simulink model "GIT_AUTO_Model_Example"  (R2019b)
settings: Solver=FixedStepDiscrete  StartTime=0.0  StopTime=10  FixedStep=0.01  RelTol=1e-3  EnableMultiTasking=on
InitFcn:
  | clear mex;
undefined symbols (not defined in the file): asbcbaseini_C, ibatini_C, k_icalpl_C, scsocini_C, stopengstmode_C, t_bmaxini_C, t_bminini_C, t_vminddstr_C, TSB_Coulomb_float, TSB_Dc_float, TSB_Pwr_float, TSB_R_float, TSB_Soc, TSB_Tbatt, TSB_Tbatt_float, TSB_value_float, TSB_Volt_float, v_bcini_C, v_bcmaxini_C
libraries: Utility_Block_Library x22, AMO_Block_Library x2
(part 3 of 5)

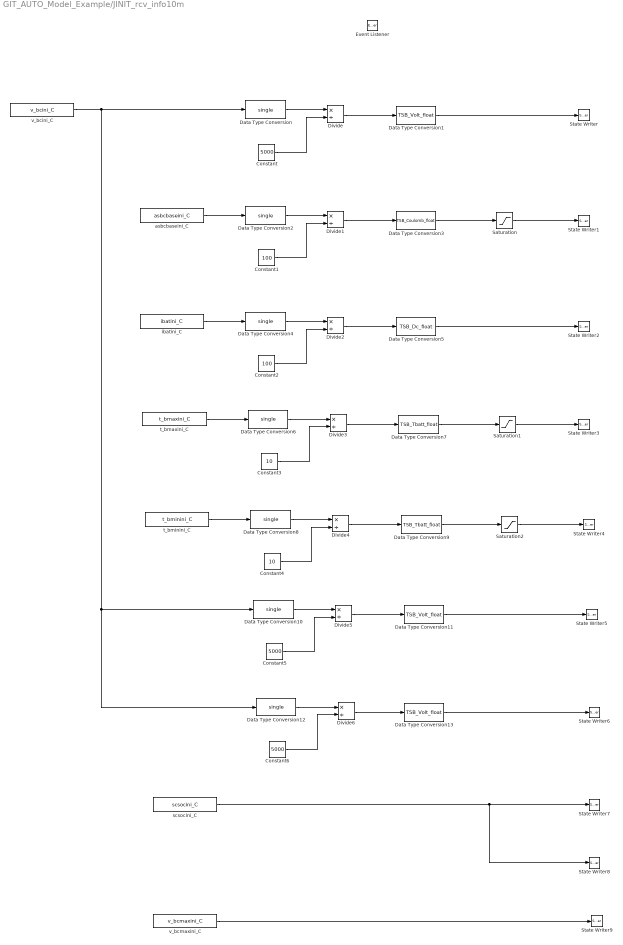
== system GIT_AUTO_Model_Example/JINIT_rcv_info10m ==
  Constant : Constant  Tag=#AMO_Lib  Value=5000  OutDataTypeStr=single
      settings: AttributesFormatString=%<Tag>\nOutDataType = %<OutDataTypeStr>
  Constant1 : Constant  Tag=#AMO_Lib  Value=100  OutDataTypeStr=single
      settings: AttributesFormatString=%<Tag>\nOutDataType = %<OutDataTypeStr>
  Constant2 : Constant  Tag=#AMO_Lib  Value=100  OutDataTypeStr=single
      settings: AttributesFormatString=%<Tag>\nOutDataType = %<OutDataTypeStr>
  Constant3 : Constant  Tag=#AMO_Lib  Value=10  OutDataTypeStr=single
      settings: AttributesFormatString=%<Tag>\nOutDataType = %<OutDataTypeStr>
  Constant4 : Constant  Tag=#AMO_Lib  Value=10  OutDataTypeStr=single
      settings: AttributesFormatString=%<Tag>\nOutDataType = %<OutDataTypeStr>
  Constant5 : Constant  Tag=#AMO_Lib  Value=5000  OutDataTypeStr=single
      settings: AttributesFormatString=%<Tag>\nOutDataType = %<OutDataTypeStr>
  Constant6 : Constant  Tag=#AMO_Lib  Value=5000  OutDataTypeStr=single
      settings: AttributesFormatString=%<Tag>\nOutDataType = %<OutDataTypeStr>
  Data Type Conversion : DataTypeConversion  Tag=#AMO_Lib  OutMin=OutMin  OutMax=OutMax  OutDataTypeStr=single  ConvertRealWorld=Stored Integer (SI)  SampleTime=SampleTime  SaturateOnIntegerOverflow=on  RndMeth=Zero  mask{OutMin=[], OutMax=[], OutDataTypeStr=single, LockScale=off, ConvertRealWorld=Stored Integer (SI), RndMeth=Zero, SaturateOnIntegerOverflow=on, SampleTime=-1}
      mask prompts: OutMin "Simulink:blkprm_prompts:OutputDesignMin"; OutMax "Simulink:blkprm_prompts:OutputDesignMax"; OutDataTypeStr "Simulink:blkprm_prompts:OUTPUT_UNIFIEDDATATYPE"; LockScale "Simulink:blkprm_prompts:LockScale"; ConvertRealWorld "Simulink:blkprm_prompts:DtypeCnvInputOutputValue"; RndMeth "Simulink:blkprm_prompts:SPP_RndMeth_ID"; SaturateOnIntegerOverflow "Simulink:blkprm_prompts:AllBlksSaturate"; SampleTime "Simulink:blkprm_prompts:AllBlksSampleTime"
      mask help:
      | 入力を出力のデータ型とスケーリングに変換します。
      |
      | この変換には 2 つの目的があります。1 つは入力と出力の実際値を等しくすることです。もう 1 つは入力と出力の整数格納値を等しくすることです。オーバーフローと量子化誤差があると、この目的を完全に達成することができません。
      settings: AttributesFormatString=%<Tag>\nOutDataType = %<OutDataTypeStr>
      mask TypeOptions OutMin: OutMin
      mask TypeOptions OutMax: OutMax
      mask TypeOptions OutDataTypeStr: OutDataTypeStr
      mask TypeOptions LockScale: LockScale
      mask TypeOptions ConvertRealWorld: ConvertRealWorld
      mask TypeOptions RndMeth: RndMeth
      mask TypeOptions SaturateOnIntegerOverflow: SaturateOnIntegerOverflow
      mask TypeOptions SampleTime: SampleTime
      mask DialogControl OutMin Prompt: 出力の最小値:
      mask DialogControl OutMax Prompt: 出力の最大値:
      mask DialogControl OutDataTypeStr Prompt: 出力データ型:
      mask DialogControl LockScale Prompt: 固定小数点ツールによる変更に対して出力データ型の設定をロックする
      mask DialogControl ConvertRealWorld Prompt: 等価な値をもつ入力と出力:
      mask DialogControl RndMeth Prompt: 整数丸めモード:
      mask DialogControl SaturateOnIntegerOverflow Prompt: 整数オーバーフローで飽和
      mask DialogControl SampleTime Prompt: サンプル時間 (継承は -1):
  Data Type Conversion1 : DataTypeConversion  Tag=#AMO_Lib  OutMin=OutMin  OutMax=OutMax  OutDataTypeStr=TSB_Volt_float  SampleTime=SampleTime  SaturateOnIntegerOverflow=on  RndMeth=Zero  mask{OutMin=[], OutMax=[], OutDataTypeStr=TSB_Volt_float, LockScale=off, ConvertRealWorld=Real World Value (RWV), RndMeth=Zero, SaturateOnIntegerOverflow=on, SampleTime=-1}
      mask prompts: OutMin "Simulink:blkprm_prompts:OutputDesignMin"; OutMax "Simulink:blkprm_prompts:OutputDesignMax"; OutDataTypeStr "Simulink:blkprm_prompts:OUTPUT_UNIFIEDDATATYPE"; LockScale "Simulink:blkprm_prompts:LockScale"; ConvertRealWorld "Simulink:blkprm_prompts:DtypeCnvInputOutputValue"; RndMeth "Simulink:blkprm_prompts:SPP_RndMeth_ID"; SaturateOnIntegerOverflow "Simulink:blkprm_prompts:AllBlksSaturate"; SampleTime "Simulink:blkprm_prompts:AllBlksSampleTime"
      mask help:
      | 入力を出力のデータ型とスケーリングに変換します。
      |
      | この変換には 2 つの目的があります。1 つは入力と出力の実際値を等しくすることです。もう 1 つは入力と出力の整数格納値を等しくすることです。オーバーフローと量子化誤差があると、この目的を完全に達成することができません。
      settings: AttributesFormatString=%<Tag>\nOutDataType = %<OutDataTypeStr>
      mask TypeOptions OutMin: OutMin
      mask TypeOptions OutMax: OutMax
      mask TypeOptions OutDataTypeStr: OutDataTypeStr
      mask TypeOptions LockScale: LockScale
      mask TypeOptions ConvertRealWorld: ConvertRealWorld
      mask TypeOptions RndMeth: RndMeth
      mask TypeOptions SaturateOnIntegerOverflow: SaturateOnIntegerOverflow
      mask TypeOptions SampleTime: SampleTime
      mask DialogControl OutMin Prompt: 出力の最小値:
      mask DialogControl OutMax Prompt: 出力の最大値:
      mask DialogControl OutDataTypeStr Prompt: 出力データ型:
      mask DialogControl LockScale Prompt: 固定小数点ツールによる変更に対して出力データ型の設定をロックする
      mask DialogControl ConvertRealWorld Prompt: 等価な値をもつ入力と出力:
      mask DialogControl RndMeth Prompt: 整数丸めモード:
      mask DialogControl SaturateOnIntegerOverflow Prompt: 整数オーバーフローで飽和
      mask DialogControl SampleTime Prompt: サンプル時間 (継承は -1):
  Data Type Conversion10 : DataTypeConversion  Tag=#AMO_Lib  OutMin=OutMin  OutMax=OutMax  OutDataTypeStr=single  ConvertRealWorld=Stored Integer (SI)  SampleTime=SampleTime  SaturateOnIntegerOverflow=on  RndMeth=Zero  mask{OutMin=[], OutMax=[], OutDataTypeStr=single, LockScale=off, ConvertRealWorld=Stored Integer (SI), RndMeth=Zero, SaturateOnIntegerOverflow=on, SampleTime=-1}
      mask prompts: OutMin "Simulink:blkprm_prompts:OutputDesignMin"; OutMax "Simulink:blkprm_prompts:OutputDesignMax"; OutDataTypeStr "Simulink:blkprm_prompts:OUTPUT_UNIFIEDDATATYPE"; LockScale "Simulink:blkprm_prompts:LockScale"; ConvertRealWorld "Simulink:blkprm_prompts:DtypeCnvInputOutputValue"; RndMeth "Simulink:blkprm_prompts:SPP_RndMeth_ID"; SaturateOnIntegerOverflow "Simulink:blkprm_prompts:AllBlksSaturate"; SampleTime "Simulink:blkprm_prompts:AllBlksSampleTime"
      mask help:
      | 入力を出力のデータ型とスケーリングに変換します。
      |
      | この変換には 2 つの目的があります。1 つは入力と出力の実際値を等しくすることです。もう 1 つは入力と出力の整数格納値を等しくすることです。オーバーフローと量子化誤差があると、この目的を完全に達成することができません。
      settings: AttributesFormatString=%<Tag>\nOutDataType = %<OutDataTypeStr>
      mask TypeOptions OutMin: OutMin
      mask TypeOptions OutMax: OutMax
      mask TypeOptions OutDataTypeStr: OutDataTypeStr
      mask TypeOptions LockScale: LockScale
      mask TypeOptions ConvertRealWorld: ConvertRealWorld
      mask TypeOptions RndMeth: RndMeth
      mask TypeOptions SaturateOnIntegerOverflow: SaturateOnIntegerOverflow
      mask TypeOptions SampleTime: SampleTime
      mask DialogControl OutMin Prompt: 出力の最小値:
      mask DialogControl OutMax Prompt: 出力の最大値:
      mask DialogControl OutDataTypeStr Prompt: 出力データ型:
      mask DialogControl LockScale Prompt: 固定小数点ツールによる変更に対して出力データ型の設定をロックする
      mask DialogControl ConvertRealWorld Prompt: 等価な値をもつ入力と出力:
      mask DialogControl RndMeth Prompt: 整数丸めモード:
      mask DialogControl SaturateOnIntegerOverflow Prompt: 整数オーバーフローで飽和
      mask DialogControl SampleTime Prompt: サンプル時間 (継承は -1):
  Data Type Conversion11 : DataTypeConversion  Tag=#AMO_Lib  OutMin=OutMin  OutMax=OutMax  OutDataTypeStr=TSB_Volt_float  SampleTime=SampleTime  SaturateOnIntegerOverflow=on  RndMeth=Zero  mask{OutMin=[], OutMax=[], OutDataTypeStr=TSB_Volt_float, LockScale=off, ConvertRealWorld=Real World Value (RWV), RndMeth=Zero, SaturateOnIntegerOverflow=on, SampleTime=-1}
      mask prompts: OutMin "Simulink:blkprm_prompts:OutputDesignMin"; OutMax "Simulink:blkprm_prompts:OutputDesignMax"; OutDataTypeStr "Simulink:blkprm_prompts:OUTPUT_UNIFIEDDATATYPE"; LockScale "Simulink:blkprm_prompts:LockScale"; ConvertRealWorld "Simulink:blkprm_prompts:DtypeCnvInputOutputValue"; RndMeth "Simulink:blkprm_prompts:SPP_RndMeth_ID"; SaturateOnIntegerOverflow "Simulink:blkprm_prompts:AllBlksSaturate"; SampleTime "Simulink:blkprm_prompts:AllBlksSampleTime"
      mask help:
      | 入力を出力のデータ型とスケーリングに変換します。
      |
      | この変換には 2 つの目的があります。1 つは入力と出力の実際値を等しくすることです。もう 1 つは入力と出力の整数格納値を等しくすることです。オーバーフローと量子化誤差があると、この目的を完全に達成することができません。
      settings: AttributesFormatString=%<Tag>\nOutDataType = %<OutDataTypeStr>
      mask TypeOptions OutMin: OutMin
      mask TypeOptions OutMax: OutMax
      mask TypeOptions OutDataTypeStr: OutDataTypeStr
      mask TypeOptions LockScale: LockScale
      mask TypeOptions ConvertRealWorld: ConvertRealWorld
      mask TypeOptions RndMeth: RndMeth
      mask TypeOptions SaturateOnIntegerOverflow: SaturateOnIntegerOverflow
      mask TypeOptions SampleTime: SampleTime
      mask DialogControl OutMin Prompt: 出力の最小値:
      mask DialogControl OutMax Prompt: 出力の最大値:
      mask DialogControl OutDataTypeStr Prompt: 出力データ型:
      mask DialogControl LockScale Prompt: 固定小数点ツールによる変更に対して出力データ型の設定をロックする
      mask DialogControl ConvertRealWorld Prompt: 等価な値をもつ入力と出力:
      mask DialogControl RndMeth Prompt: 整数丸めモード:
      mask DialogControl SaturateOnIntegerOverflow Prompt: 整数オーバーフローで飽和
      mask DialogControl SampleTime Prompt: サンプル時間 (継承は -1):
  Data Type Conversion12 : DataTypeConversion  Tag=#AMO_Lib  OutMin=OutMin  OutMax=OutMax  OutDataTypeStr=single  ConvertRealWorld=Stored Integer (SI)  SampleTime=SampleTime  SaturateOnIntegerOverflow=on  RndMeth=Zero  mask{OutMin=[], OutMax=[], OutDataTypeStr=single, LockScale=off, ConvertRealWorld=Stored Integer (SI), RndMeth=Zero, SaturateOnIntegerOverflow=on, SampleTime=-1}
      mask prompts: OutMin "Simulink:blkprm_prompts:OutputDesignMin"; OutMax "Simulink:blkprm_prompts:OutputDesignMax"; OutDataTypeStr "Simulink:blkprm_prompts:OUTPUT_UNIFIEDDATATYPE"; LockScale "Simulink:blkprm_prompts:LockScale"; ConvertRealWorld "Simulink:blkprm_prompts:DtypeCnvInputOutputValue"; RndMeth "Simulink:blkprm_prompts:SPP_RndMeth_ID"; SaturateOnIntegerOverflow "Simulink:blkprm_prompts:AllBlksSaturate"; SampleTime "Simulink:blkprm_prompts:AllBlksSampleTime"
      mask help:
      | 入力を出力のデータ型とスケーリングに変換します。
      |
      | この変換には 2 つの目的があります。1 つは入力と出力の実際値を等しくすることです。もう 1 つは入力と出力の整数格納値を等しくすることです。オーバーフローと量子化誤差があると、この目的を完全に達成することができません。
      settings: AttributesFormatString=%<Tag>\nOutDataType = %<OutDataTypeStr>
      mask TypeOptions OutMin: OutMin
      mask TypeOptions OutMax: OutMax
      mask TypeOptions OutDataTypeStr: OutDataTypeStr
      mask TypeOptions LockScale: LockScale
      mask TypeOptions ConvertRealWorld: ConvertRealWorld
      mask TypeOptions RndMeth: RndMeth
      mask TypeOptions SaturateOnIntegerOverflow: SaturateOnIntegerOverflow
      mask TypeOptions SampleTime: SampleTime
      mask DialogControl OutMin Prompt: 出力の最小値:
      mask DialogControl OutMax Prompt: 出力の最大値:
      mask DialogControl OutDataTypeStr Prompt: 出力データ型:
      mask DialogControl LockScale Prompt: 固定小数点ツールによる変更に対して出力データ型の設定をロックする
      mask DialogControl ConvertRealWorld Prompt: 等価な値をもつ入力と出力:
      mask DialogControl RndMeth Prompt: 整数丸めモード:
      mask DialogControl SaturateOnIntegerOverflow Prompt: 整数オーバーフローで飽和
      mask DialogControl SampleTime Prompt: サンプル時間 (継承は -1):
  Data Type Conversion13 : DataTypeConversion  Tag=#AMO_Lib  OutMin=OutMin  OutMax=OutMax  OutDataTypeStr=TSB_Volt_float  SampleTime=SampleTime  SaturateOnIntegerOverflow=on  RndMeth=Zero  mask{OutMin=[], OutMax=[], OutDataTypeStr=TSB_Volt_float, LockScale=off, ConvertRealWorld=Real World Value (RWV), RndMeth=Zero, SaturateOnIntegerOverflow=on, SampleTime=-1}
      mask prompts: OutMin "Simulink:blkprm_prompts:OutputDesignMin"; OutMax "Simulink:blkprm_prompts:OutputDesignMax"; OutDataTypeStr "Simulink:blkprm_prompts:OUTPUT_UNIFIEDDATATYPE"; LockScale "Simulink:blkprm_prompts:LockScale"; ConvertRealWorld "Simulink:blkprm_prompts:DtypeCnvInputOutputValue"; RndMeth "Simulink:blkprm_prompts:SPP_RndMeth_ID"; SaturateOnIntegerOverflow "Simulink:blkprm_prompts:AllBlksSaturate"; SampleTime "Simulink:blkprm_prompts:AllBlksSampleTime"
      mask help:
      | 入力を出力のデータ型とスケーリングに変換します。
      |
      | この変換には 2 つの目的があります。1 つは入力と出力の実際値を等しくすることです。もう 1 つは入力と出力の整数格納値を等しくすることです。オーバーフローと量子化誤差があると、この目的を完全に達成することができません。
      settings: AttributesFormatString=%<Tag>\nOutDataType = %<OutDataTypeStr>
      mask TypeOptions OutMin: OutMin
      mask TypeOptions OutMax: OutMax
      mask TypeOptions OutDataTypeStr: OutDataTypeStr
      mask TypeOptions LockScale: LockScale
      mask TypeOptions ConvertRealWorld: ConvertRealWorld
      mask TypeOptions RndMeth: RndMeth
      mask TypeOptions SaturateOnIntegerOverflow: SaturateOnIntegerOverflow
      mask TypeOptions SampleTime: SampleTime
      mask DialogControl OutMin Prompt: 出力の最小値:
      mask DialogControl OutMax Prompt: 出力の最大値:
      mask DialogControl OutDataTypeStr Prompt: 出力データ型:
      mask DialogControl LockScale Prompt: 固定小数点ツールによる変更に対して出力データ型の設定をロックする
      mask DialogControl ConvertRealWorld Prompt: 等価な値をもつ入力と出力:
      mask DialogControl RndMeth Prompt: 整数丸めモード:
      mask DialogControl SaturateOnIntegerOverflow Prompt: 整数オーバーフローで飽和
      mask DialogControl SampleTime Prompt: サンプル時間 (継承は -1):
  Data Type Conversion2 : DataTypeConversion  Tag=#AMO_Lib  OutMin=OutMin  OutMax=OutMax  OutDataTypeStr=single  ConvertRealWorld=Stored Integer (SI)  SampleTime=SampleTime  SaturateOnIntegerOverflow=on  RndMeth=Zero  mask{OutMin=[], OutMax=[], OutDataTypeStr=single, LockScale=off, ConvertRealWorld=Stored Integer (SI), RndMeth=Zero, SaturateOnIntegerOverflow=on, SampleTime=-1}
      mask prompts: OutMin "Simulink:blkprm_prompts:OutputDesignMin"; OutMax "Simulink:blkprm_prompts:OutputDesignMax"; OutDataTypeStr "Simulink:blkprm_prompts:OUTPUT_UNIFIEDDATATYPE"; LockScale "Simulink:blkprm_prompts:LockScale"; ConvertRealWorld "Simulink:blkprm_prompts:DtypeCnvInputOutputValue"; RndMeth "Simulink:blkprm_prompts:SPP_RndMeth_ID"; SaturateOnIntegerOverflow "Simulink:blkprm_prompts:AllBlksSaturate"; SampleTime "Simulink:blkprm_prompts:AllBlksSampleTime"
      mask help:
      | 入力を出力のデータ型とスケーリングに変換します。
      |
      | この変換には 2 つの目的があります。1 つは入力と出力の実際値を等しくすることです。もう 1 つは入力と出力の整数格納値を等しくすることです。オーバーフローと量子化誤差があると、この目的を完全に達成することができません。
      settings: AttributesFormatString=%<Tag>\nOutDataType = %<OutDataTypeStr>
      mask TypeOptions OutMin: OutMin
      mask TypeOptions OutMax: OutMax
      mask TypeOptions OutDataTypeStr: OutDataTypeStr
      mask TypeOptions LockScale: LockScale
      mask TypeOptions ConvertRealWorld: ConvertRealWorld
      mask TypeOptions RndMeth: RndMeth
      mask TypeOptions SaturateOnIntegerOverflow: SaturateOnIntegerOverflow
      mask TypeOptions SampleTime: SampleTime
      mask DialogControl OutMin Prompt: 出力の最小値:
      mask DialogControl OutMax Prompt: 出力の最大値:
      mask DialogControl OutDataTypeStr Prompt: 出力データ型:
      mask DialogControl LockScale Prompt: 固定小数点ツールによる変更に対して出力データ型の設定をロックする
      mask DialogControl ConvertRealWorld Prompt: 等価な値をもつ入力と出力:
      mask DialogControl RndMeth Prompt: 整数丸めモード:
      mask DialogControl SaturateOnIntegerOverflow Prompt: 整数オーバーフローで飽和
      mask DialogControl SampleTime Prompt: サンプル時間 (継承は -1):
  Data Type Conversion3 : DataTypeConversion  Tag=#AMO_Lib  OutMin=OutMin  OutMax=OutMax  OutDataTypeStr=TSB_Coulomb_float  SampleTime=SampleTime  SaturateOnIntegerOverflow=on  RndMeth=Zero  mask{OutMin=[], OutMax=[], OutDataTypeStr=TSB_Coulomb_float, LockScale=off, ConvertRealWorld=Real World Value (RWV), RndMeth=Zero, SaturateOnIntegerOverflow=on, SampleTime=-1}
      mask prompts: OutMin "Simulink:blkprm_prompts:OutputDesignMin"; OutMax "Simulink:blkprm_prompts:OutputDesignMax"; OutDataTypeStr "Simulink:blkprm_prompts:OUTPUT_UNIFIEDDATATYPE"; LockScale "Simulink:blkprm_prompts:LockScale"; ConvertRealWorld "Simulink:blkprm_prompts:DtypeCnvInputOutputValue"; RndMeth "Simulink:blkprm_prompts:SPP_RndMeth_ID"; SaturateOnIntegerOverflow "Simulink:blkprm_prompts:AllBlksSaturate"; SampleTime "Simulink:blkprm_prompts:AllBlksSampleTime"
      mask help:
      | 入力を出力のデータ型とスケーリングに変換します。
      |
      | この変換には 2 つの目的があります。1 つは入力と出力の実際値を等しくすることです。もう 1 つは入力と出力の整数格納値を等しくすることです。オーバーフローと量子化誤差があると、この目的を完全に達成することができません。
      settings: AttributesFormatString=%<Tag>\nOutDataType = %<OutDataTypeStr>
      mask TypeOptions OutMin: OutMin
      mask TypeOptions OutMax: OutMax
      mask TypeOptions OutDataTypeStr: OutDataTypeStr
      mask TypeOptions LockScale: LockScale
      mask TypeOptions ConvertRealWorld: ConvertRealWorld
      mask TypeOptions RndMeth: RndMeth
      mask TypeOptions SaturateOnIntegerOverflow: SaturateOnIntegerOverflow
      mask TypeOptions SampleTime: SampleTime
      mask DialogControl OutMin Prompt: 出力の最小値:
      mask DialogControl OutMax Prompt: 出力の最大値:
      mask DialogControl OutDataTypeStr Prompt: 出力データ型:
      mask DialogControl LockScale Prompt: 固定小数点ツールによる変更に対して出力データ型の設定をロックする
      mask DialogControl ConvertRealWorld Prompt: 等価な値をもつ入力と出力:
      mask DialogControl RndMeth Prompt: 整数丸めモード:
      mask DialogControl SaturateOnIntegerOverflow Prompt: 整数オーバーフローで飽和
      mask DialogControl SampleTime Prompt: サンプル時間 (継承は -1):
  Data Type Conversion4 : DataTypeConversion  Tag=#AMO_Lib  OutMin=OutMin  OutMax=OutMax  OutDataTypeStr=single  ConvertRealWorld=Stored Integer (SI)  SampleTime=SampleTime  SaturateOnIntegerOverflow=on  RndMeth=Zero  mask{OutMin=[], OutMax=[], OutDataTypeStr=single, LockScale=off, ConvertRealWorld=Stored Integer (SI), RndMeth=Zero, SaturateOnIntegerOverflow=on, SampleTime=-1}
      mask prompts: OutMin "Simulink:blkprm_prompts:OutputDesignMin"; OutMax "Simulink:blkprm_prompts:OutputDesignMax"; OutDataTypeStr "Simulink:blkprm_prompts:OUTPUT_UNIFIEDDATATYPE"; LockScale "Simulink:blkprm_prompts:LockScale"; ConvertRealWorld "Simulink:blkprm_prompts:DtypeCnvInputOutputValue"; RndMeth "Simulink:blkprm_prompts:SPP_RndMeth_ID"; SaturateOnIntegerOverflow "Simulink:blkprm_prompts:AllBlksSaturate"; SampleTime "Simulink:blkprm_prompts:AllBlksSampleTime"
      mask help:
      | 入力を出力のデータ型とスケーリングに変換します。
      |
      | この変換には 2 つの目的があります。1 つは入力と出力の実際値を等しくすることです。もう 1 つは入力と出力の整数格納値を等しくすることです。オーバーフローと量子化誤差があると、この目的を完全に達成することができません。
      settings: AttributesFormatString=%<Tag>\nOutDataType = %<OutDataTypeStr>
      mask TypeOptions OutMin: OutMin
      mask TypeOptions OutMax: OutMax
      mask TypeOptions OutDataTypeStr: OutDataTypeStr
      mask TypeOptions LockScale: LockScale
      mask TypeOptions ConvertRealWorld: ConvertRealWorld
      mask TypeOptions RndMeth: RndMeth
      mask TypeOptions SaturateOnIntegerOverflow: SaturateOnIntegerOverflow
      mask TypeOptions SampleTime: SampleTime
      mask DialogControl OutMin Prompt: 出力の最小値:
      mask DialogControl OutMax Prompt: 出力の最大値:
      mask DialogControl OutDataTypeStr Prompt: 出力データ型:
      mask DialogControl LockScale Prompt: 固定小数点ツールによる変更に対して出力データ型の設定をロックする
      mask DialogControl ConvertRealWorld Prompt: 等価な値をもつ入力と出力:
      mask DialogControl RndMeth Prompt: 整数丸めモード:
      mask DialogControl SaturateOnIntegerOverflow Prompt: 整数オーバーフローで飽和
      mask DialogControl SampleTime Prompt: サンプル時間 (継承は -1):
  Data Type Conversion5 : DataTypeConversion  Tag=#AMO_Lib  OutMin=OutMin  OutMax=OutMax  OutDataTypeStr=TSB_Dc_float  SampleTime=SampleTime  SaturateOnIntegerOverflow=on  RndMeth=Zero  mask{OutMin=[], OutMax=[], OutDataTypeStr=TSB_Dc_float, LockScale=off, ConvertRealWorld=Real World Value (RWV), RndMeth=Zero, SaturateOnIntegerOverflow=on, SampleTime=-1}
      mask prompts: OutMin "Simulink:blkprm_prompts:OutputDesignMin"; OutMax "Simulink:blkprm_prompts:OutputDesignMax"; OutDataTypeStr "Simulink:blkprm_prompts:OUTPUT_UNIFIEDDATATYPE"; LockScale "Simulink:blkprm_prompts:LockScale"; ConvertRealWorld "Simulink:blkprm_prompts:DtypeCnvInputOutputValue"; RndMeth "Simulink:blkprm_prompts:SPP_RndMeth_ID"; SaturateOnIntegerOverflow "Simulink:blkprm_prompts:AllBlksSaturate"; SampleTime "Simulink:blkprm_prompts:AllBlksSampleTime"
      mask help:
      | 入力を出力のデータ型とスケーリングに変換します。
      |
      | この変換には 2 つの目的があります。1 つは入力と出力の実際値を等しくすることです。もう 1 つは入力と出力の整数格納値を等しくすることです。オーバーフローと量子化誤差があると、この目的を完全に達成することができません。
      settings: AttributesFormatString=%<Tag>\nOutDataType = %<OutDataTypeStr>
      mask TypeOptions OutMin: OutMin
      mask TypeOptions OutMax: OutMax
      mask TypeOptions OutDataTypeStr: OutDataTypeStr
      mask TypeOptions LockScale: LockScale
      mask TypeOptions ConvertRealWorld: ConvertRealWorld
      mask TypeOptions RndMeth: RndMeth
      mask TypeOptions SaturateOnIntegerOverflow: SaturateOnIntegerOverflow
      mask TypeOptions SampleTime: SampleTime
      mask DialogControl OutMin Prompt: 出力の最小値:
      mask DialogControl OutMax Prompt: 出力の最大値:
      mask DialogControl OutDataTypeStr Prompt: 出力データ型:
      mask DialogControl LockScale Prompt: 固定小数点ツールによる変更に対して出力データ型の設定をロックする
      mask DialogControl ConvertRealWorld Prompt: 等価な値をもつ入力と出力:
      mask DialogControl RndMeth Prompt: 整数丸めモード:
      mask DialogControl SaturateOnIntegerOverflow Prompt: 整数オーバーフローで飽和
      mask DialogControl SampleTime Prompt: サンプル時間 (継承は -1):
  Data Type Conversion6 : DataTypeConversion  Tag=#AMO_Lib  OutMin=OutMin  OutMax=OutMax  OutDataTypeStr=single  ConvertRealWorld=Stored Integer (SI)  SampleTime=SampleTime  SaturateOnIntegerOverflow=on  RndMeth=Zero  mask{OutMin=[], OutMax=[], OutDataTypeStr=single, LockScale=off, ConvertRealWorld=Stored Integer (SI), RndMeth=Zero, SaturateOnIntegerOverflow=on, SampleTime=-1}
      mask prompts: OutMin "Simulink:blkprm_prompts:OutputDesignMin"; OutMax "Simulink:blkprm_prompts:OutputDesignMax"; OutDataTypeStr "Simulink:blkprm_prompts:OUTPUT_UNIFIEDDATATYPE"; LockScale "Simulink:blkprm_prompts:LockScale"; ConvertRealWorld "Simulink:blkprm_prompts:DtypeCnvInputOutputValue"; RndMeth "Simulink:blkprm_prompts:SPP_RndMeth_ID"; SaturateOnIntegerOverflow "Simulink:blkprm_prompts:AllBlksSaturate"; SampleTime "Simulink:blkprm_prompts:AllBlksSampleTime"
      mask help:
      | 入力を出力のデータ型とスケーリングに変換します。
      |
      | この変換には 2 つの目的があります。1 つは入力と出力の実際値を等しくすることです。もう 1 つは入力と出力の整数格納値を等しくすることです。オーバーフローと量子化誤差があると、この目的を完全に達成することができません。
      settings: AttributesFormatString=%<Tag>\nOutDataType = %<OutDataTypeStr>
      mask TypeOptions OutMin: OutMin
      mask TypeOptions OutMax: OutMax
      mask TypeOptions OutDataTypeStr: OutDataTypeStr
      mask TypeOptions LockScale: LockScale
      mask TypeOptions ConvertRealWorld: ConvertRealWorld
      mask TypeOptions RndMeth: RndMeth
      mask TypeOptions SaturateOnIntegerOverflow: SaturateOnIntegerOverflow
      mask TypeOptions SampleTime: SampleTime
      mask DialogControl OutMin Prompt: 出力の最小値:
      mask DialogControl OutMax Prompt: 出力の最大値:
      mask DialogControl OutDataTypeStr Prompt: 出力データ型:
      mask DialogControl LockScale Prompt: 固定小数点ツールによる変更に対して出力データ型の設定をロックする
      mask DialogControl ConvertRealWorld Prompt: 等価な値をもつ入力と出力:
      mask DialogControl RndMeth Prompt: 整数丸めモード:
      mask DialogControl SaturateOnIntegerOverflow Prompt: 整数オーバーフローで飽和
      mask DialogControl SampleTime Prompt: サンプル時間 (継承は -1):
  Data Type Conversion7 : DataTypeConversion  Tag=#AMO_Lib  OutMin=OutMin  OutMax=OutMax  OutDataTypeStr=TSB_Tbatt_float  SampleTime=SampleTime  SaturateOnIntegerOverflow=on  RndMeth=Zero  mask{OutMin=[], OutMax=[], OutDataTypeStr=TSB_Tbatt_float, LockScale=off, ConvertRealWorld=Real World Value (RWV), RndMeth=Zero, SaturateOnIntegerOverflow=on, SampleTime=-1}
      mask prompts: OutMin "Simulink:blkprm_prompts:OutputDesignMin"; OutMax "Simulink:blkprm_prompts:OutputDesignMax"; OutDataTypeStr "Simulink:blkprm_prompts:OUTPUT_UNIFIEDDATATYPE"; LockScale "Simulink:blkprm_prompts:LockScale"; ConvertRealWorld "Simulink:blkprm_prompts:DtypeCnvInputOutputValue"; RndMeth "Simulink:blkprm_prompts:SPP_RndMeth_ID"; SaturateOnIntegerOverflow "Simulink:blkprm_prompts:AllBlksSaturate"; SampleTime "Simulink:blkprm_prompts:AllBlksSampleTime"
      mask help:
      | 入力を出力のデータ型とスケーリングに変換します。
      |
      | この変換には 2 つの目的があります。1 つは入力と出力の実際値を等しくすることです。もう 1 つは入力と出力の整数格納値を等しくすることです。オーバーフローと量子化誤差があると、この目的を完全に達成することができません。
      settings: AttributesFormatString=%<Tag>\nOutDataType = %<OutDataTypeStr>
      mask TypeOptions OutMin: OutMin
      mask TypeOptions OutMax: OutMax
      mask TypeOptions OutDataTypeStr: OutDataTypeStr
      mask TypeOptions LockScale: LockScale
      mask TypeOptions ConvertRealWorld: ConvertRealWorld
      mask TypeOptions RndMeth: RndMeth
      mask TypeOptions SaturateOnIntegerOverflow: SaturateOnIntegerOverflow
      mask TypeOptions SampleTime: SampleTime
      mask DialogControl OutMin Prompt: 出力の最小値:
      mask DialogControl OutMax Prompt: 出力の最大値:
      mask DialogControl OutDataTypeStr Prompt: 出力データ型:
      mask DialogControl LockScale Prompt: 固定小数点ツールによる変更に対して出力データ型の設定をロックする
      mask DialogControl ConvertRealWorld Prompt: 等価な値をもつ入力と出力:
      mask DialogControl RndMeth Prompt: 整数丸めモード:
      mask DialogControl SaturateOnIntegerOverflow Prompt: 整数オーバーフローで飽和
      mask DialogControl SampleTime Prompt: サンプル時間 (継承は -1):
  Data Type Conversion8 : DataTypeConversion  Tag=#AMO_Lib  OutMin=OutMin  OutMax=OutMax  OutDataTypeStr=single  ConvertRealWorld=Stored Integer (SI)  SampleTime=SampleTime  SaturateOnIntegerOverflow=on  RndMeth=Zero  mask{OutMin=[], OutMax=[], OutDataTypeStr=single, LockScale=off, ConvertRealWorld=Stored Integer (SI), RndMeth=Zero, SaturateOnIntegerOverflow=on, SampleTime=-1}
      mask prompts: OutMin "Simulink:blkprm_prompts:OutputDesignMin"; OutMax "Simulink:blkprm_prompts:OutputDesignMax"; OutDataTypeStr "Simulink:blkprm_prompts:OUTPUT_UNIFIEDDATATYPE"; LockScale "Simulink:blkprm_prompts:LockScale"; ConvertRealWorld "Simulink:blkprm_prompts:DtypeCnvInputOutputValue"; RndMeth "Simulink:blkprm_prompts:SPP_RndMeth_ID"; SaturateOnIntegerOverflow "Simulink:blkprm_prompts:AllBlksSaturate"; SampleTime "Simulink:blkprm_prompts:AllBlksSampleTime"
      mask help:
      | 入力を出力のデータ型とスケーリングに変換します。
      |
      | この変換には 2 つの目的があります。1 つは入力と出力の実際値を等しくすることです。もう 1 つは入力と出力の整数格納値を等しくすることです。オーバーフローと量子化誤差があると、この目的を完全に達成することができません。
      settings: AttributesFormatString=%<Tag>\nOutDataType = %<OutDataTypeStr>
      mask TypeOptions OutMin: OutMin
      mask TypeOptions OutMax: OutMax
      mask TypeOptions OutDataTypeStr: OutDataTypeStr
      mask TypeOptions LockScale: LockScale
      mask TypeOptions ConvertRealWorld: ConvertRealWorld
      mask TypeOptions RndMeth: RndMeth
      mask TypeOptions SaturateOnIntegerOverflow: SaturateOnIntegerOverflow
      mask TypeOptions SampleTime: SampleTime
      mask DialogControl OutMin Prompt: 出力の最小値:
      mask DialogControl OutMax Prompt: 出力の最大値:
      mask DialogControl OutDataTypeStr Prompt: 出力データ型:
      mask DialogControl LockScale Prompt: 固定小数点ツールによる変更に対して出力データ型の設定をロックする
      mask DialogControl ConvertRealWorld Prompt: 等価な値をもつ入力と出力:
      mask DialogControl RndMeth Prompt: 整数丸めモード:
      mask DialogControl SaturateOnIntegerOverflow Prompt: 整数オーバーフローで飽和
      mask DialogControl SampleTime Prompt: サンプル時間 (継承は -1):
  Data Type Conversion9 : DataTypeConversion  Tag=#AMO_Lib  OutMin=OutMin  OutMax=OutMax  OutDataTypeStr=TSB_Tbatt_float  SampleTime=SampleTime  SaturateOnIntegerOverflow=on  RndMeth=Zero  mask{OutMin=[], OutMax=[], OutDataTypeStr=TSB_Tbatt_float, LockScale=off, ConvertRealWorld=Real World Value (RWV), RndMeth=Zero, SaturateOnIntegerOverflow=on, SampleTime=-1}
      mask prompts: OutMin "Simulink:blkprm_prompts:OutputDesignMin"; OutMax "Simulink:blkprm_prompts:OutputDesignMax"; OutDataTypeStr "Simulink:blkprm_prompts:OUTPUT_UNIFIEDDATATYPE"; LockScale "Simulink:blkprm_prompts:LockScale"; ConvertRealWorld "Simulink:blkprm_prompts:DtypeCnvInputOutputValue"; RndMeth "Simulink:blkprm_prompts:SPP_RndMeth_ID"; SaturateOnIntegerOverflow "Simulink:blkprm_prompts:AllBlksSaturate"; SampleTime "Simulink:blkprm_prompts:AllBlksSampleTime"
      mask help:
      | 入力を出力のデータ型とスケーリングに変換します。
      |
      | この変換には 2 つの目的があります。1 つは入力と出力の実際値を等しくすることです。もう 1 つは入力と出力の整数格納値を等しくすることです。オーバーフローと量子化誤差があると、この目的を完全に達成することができません。
      settings: AttributesFormatString=%<Tag>\nOutDataType = %<OutDataTypeStr>
      mask TypeOptions OutMin: OutMin
      mask TypeOptions OutMax: OutMax
      mask TypeOptions OutDataTypeStr: OutDataTypeStr
      mask TypeOptions LockScale: LockScale
      mask TypeOptions ConvertRealWorld: ConvertRealWorld
      mask TypeOptions RndMeth: RndMeth
      mask TypeOptions SaturateOnIntegerOverflow: SaturateOnIntegerOverflow
      mask TypeOptions SampleTime: SampleTime
      mask DialogControl OutMin Prompt: 出力の最小値:
      mask DialogControl OutMax Prompt: 出力の最大値:
      mask DialogControl OutDataTypeStr Prompt: 出力データ型:
      mask DialogControl LockScale Prompt: 固定小数点ツールによる変更に対して出力データ型の設定をロックする
      mask DialogControl ConvertRealWorld Prompt: 等価な値をもつ入力と出力:
      mask DialogControl RndMeth Prompt: 整数丸めモード:
      mask DialogControl SaturateOnIntegerOverflow Prompt: 整数オーバーフローで飽和
      mask DialogControl SampleTime Prompt: サンプル時間 (継承は -1):
  Divide : Product  Tag=#AMO_Lib  Inputs=*/  CollapseDim=CollapseDim  OutMin=OutMin  OutMax=OutMax  SampleTime=SampleTime  SaturateOnIntegerOverflow=on  RndMeth=Zero  mask{Inputs=*/, Multiplication=Element-wise(.*), CollapseMode=All dimensions, CollapseDim=1, SampleTime=-1, InputSameDT=off, OutMin=[], OutMax=[], OutDataTypeStr=Inherit: Inherit via internal rule, LockScale=off, RndMeth=Zero, SaturateOnIntegerOverflow=on}
      mask prompts: Inputs "Simulink:blkprm_prompts:ProdNumInputs"; Multiplication "Simulink:blkprm_prompts:ProdMultiplication"; CollapseMode "Simulink:blkprm_prompts:ProdOperationType"; CollapseDim "Simulink:blkprm_prompts:ProdOperationDim"; SampleTime "Simulink:blkprm_prompts:AllBlksSampleTime"; InputSameDT "Simulink:blkprm_prompts:InputSameDT"; OutMin "Simulink:blkprm_prompts:OutputDesignMin"; OutMax "Simulink:blkprm_prompts:OutputDesignMax"; OutDataTypeStr "Simulink:blkprm_prompts:OUTPUT_UNIFIEDDATATYPE"; LockScale "Simulink:blkprm_prompts:LockScale"; RndMeth "Simulink:blkprm_prompts:SPP_RndMeth_ID"; SaturateOnIntegerOverflow "Simulink:blkprm_prompts:AllBlksSaturate"
      mask help:
      | 入力を乗算または除算します。要素単位、または行列の乗算を選択し、以下のいずれかを指定してください:
      |  a) 各入力端子に対して * または /。たとえば、**/* は演算 'u1*u2/u3*u4' を実行します。
      |  b) 乗算を行う入力端子の数を指定するスカラー値。たとえば、2 は演算 'u1*u2' を実行します。
      |
      | 1 つの入力端子のみがあり、乗算パラメーターが要素単位 (.*) に設定されている場合、1 つの * または / は、指定した演算を各要素に適用します。しかし、乗算パラメーターが行列 (*) に設定されている場合、1 つの * は行列の乗算を出力し、1 つの / は逆行列を出力します。
      settings: AttributesFormatString=%<Tag>\nOutDataType = %<OutDataTypeStr>
      mask TypeOptions Inputs: Inputs
      mask TypeOptions Multiplication: Multiplication
      mask TypeOptions CollapseMode: CollapseMode
      mask TypeOptions CollapseDim: CollapseDim
      mask TypeOptions SampleTime: SampleTime
      mask TypeOptions InputSameDT: InputSameDT
      mask TypeOptions OutMin: OutMin
      mask TypeOptions OutMax: OutMax
      mask TypeOptions OutDataTypeStr: OutDataTypeStr
      mask TypeOptions LockScale: LockScale
      mask TypeOptions RndMeth: RndMeth
      mask TypeOptions SaturateOnIntegerOverflow: SaturateOnIntegerOverflow
      mask DialogControl Container7 Prompt: メイン
      mask DialogControl Inputs Prompt: 入力数:
      mask DialogControl Multiplication Prompt: 乗算:
      mask DialogControl CollapseMode Prompt: 乗算範囲:
      mask DialogControl CollapseDim Prompt: 次元:
      mask DialogControl SampleTime Prompt: サンプル時間 (継承は -1):
      mask DialogControl Container8 Prompt: 信号属性
      mask DialogControl InputSameDT Prompt: すべての入力が同じデータ型をもつ
      mask DialogControl OutMin Prompt: 出力の最小値:
      mask DialogControl OutMax Prompt: 出力の最大値:
      mask DialogControl OutDataTypeStr Prompt: 出力データ型:
      mask DialogControl LockScale Prompt: 固定小数点ツールによる変更に対して出力データ型の設定をロックする
      mask DialogControl RndMeth Prompt: 整数丸めモード:
      mask DialogControl SaturateOnIntegerOverflow Prompt: 整数オーバーフローで飽和
  Divide1 : Product  Tag=#AMO_Lib  Inputs=*/  CollapseDim=CollapseDim  OutMin=OutMin  OutMax=OutMax  SampleTime=SampleTime  SaturateOnIntegerOverflow=on  RndMeth=Zero  mask{Inputs=*/, Multiplication=Element-wise(.*), CollapseMode=All dimensions, CollapseDim=1, SampleTime=-1, InputSameDT=off, OutMin=[], OutMax=[], OutDataTypeStr=Inherit: Inherit via internal rule, LockScale=off, RndMeth=Zero, SaturateOnIntegerOverflow=on}
      mask prompts: Inputs "Simulink:blkprm_prompts:ProdNumInputs"; Multiplication "Simulink:blkprm_prompts:ProdMultiplication"; CollapseMode "Simulink:blkprm_prompts:ProdOperationType"; CollapseDim "Simulink:blkprm_prompts:ProdOperationDim"; SampleTime "Simulink:blkprm_prompts:AllBlksSampleTime"; InputSameDT "Simulink:blkprm_prompts:InputSameDT"; OutMin "Simulink:blkprm_prompts:OutputDesignMin"; OutMax "Simulink:blkprm_prompts:OutputDesignMax"; OutDataTypeStr "Simulink:blkprm_prompts:OUTPUT_UNIFIEDDATATYPE"; LockScale "Simulink:blkprm_prompts:LockScale"; RndMeth "Simulink:blkprm_prompts:SPP_RndMeth_ID"; SaturateOnIntegerOverflow "Simulink:blkprm_prompts:AllBlksSaturate"
      mask help:
      | 入力を乗算または除算します。要素単位、または行列の乗算を選択し、以下のいずれかを指定してください:
      |  a) 各入力端子に対して * または /。たとえば、**/* は演算 'u1*u2/u3*u4' を実行します。
      |  b) 乗算を行う入力端子の数を指定するスカラー値。たとえば、2 は演算 'u1*u2' を実行します。
      |
      | 1 つの入力端子のみがあり、乗算パラメーターが要素単位 (.*) に設定されている場合、1 つの * または / は、指定した演算を各要素に適用します。しかし、乗算パラメーターが行列 (*) に設定されている場合、1 つの * は行列の乗算を出力し、1 つの / は逆行列を出力します。
      settings: AttributesFormatString=%<Tag>\nOutDataType = %<OutDataTypeStr>
      mask TypeOptions Inputs: Inputs
      mask TypeOptions Multiplication: Multiplication
      mask TypeOptions CollapseMode: CollapseMode
      mask TypeOptions CollapseDim: CollapseDim
      mask TypeOptions SampleTime: SampleTime
      mask TypeOptions InputSameDT: InputSameDT
      mask TypeOptions OutMin: OutMin
      mask TypeOptions OutMax: OutMax
      mask TypeOptions OutDataTypeStr: OutDataTypeStr
      mask TypeOptions LockScale: LockScale
      mask TypeOptions RndMeth: RndMeth
      mask TypeOptions SaturateOnIntegerOverflow: SaturateOnIntegerOverflow
      mask DialogControl Container7 Prompt: メイン
      mask DialogControl Inputs Prompt: 入力数:
      mask DialogControl Multiplication Prompt: 乗算:
      mask DialogControl CollapseMode Prompt: 乗算範囲:
      mask DialogControl CollapseDim Prompt: 次元:
      mask DialogControl SampleTime Prompt: サンプル時間 (継承は -1):
      mask DialogControl Container8 Prompt: 信号属性
      mask DialogControl InputSameDT Prompt: すべての入力が同じデータ型をもつ
      mask DialogControl OutMin Prompt: 出力の最小値:
      mask DialogControl OutMax Prompt: 出力の最大値:
      mask DialogControl OutDataTypeStr Prompt: 出力データ型:
      mask DialogControl LockScale Prompt: 固定小数点ツールによる変更に対して出力データ型の設定をロックする
      mask DialogControl RndMeth Prompt: 整数丸めモード:
      mask DialogControl SaturateOnIntegerOverflow Prompt: 整数オーバーフローで飽和
  Divide2 : Product  Tag=#AMO_Lib  Inputs=*/  CollapseDim=CollapseDim  OutMin=OutMin  OutMax=OutMax  SampleTime=SampleTime  SaturateOnIntegerOverflow=on  RndMeth=Zero  mask{Inputs=*/, Multiplication=Element-wise(.*), CollapseMode=All dimensions, CollapseDim=1, SampleTime=-1, InputSameDT=off, OutMin=[], OutMax=[], OutDataTypeStr=Inherit: Inherit via internal rule, LockScale=off, RndMeth=Zero, SaturateOnIntegerOverflow=on}
      mask prompts: Inputs "Simulink:blkprm_prompts:ProdNumInputs"; Multiplication "Simulink:blkprm_prompts:ProdMultiplication"; CollapseMode "Simulink:blkprm_prompts:ProdOperationType"; CollapseDim "Simulink:blkprm_prompts:ProdOperationDim"; SampleTime "Simulink:blkprm_prompts:AllBlksSampleTime"; InputSameDT "Simulink:blkprm_prompts:InputSameDT"; OutMin "Simulink:blkprm_prompts:OutputDesignMin"; OutMax "Simulink:blkprm_prompts:OutputDesignMax"; OutDataTypeStr "Simulink:blkprm_prompts:OUTPUT_UNIFIEDDATATYPE"; LockScale "Simulink:blkprm_prompts:LockScale"; RndMeth "Simulink:blkprm_prompts:SPP_RndMeth_ID"; SaturateOnIntegerOverflow "Simulink:blkprm_prompts:AllBlksSaturate"
      mask help:
      | 入力を乗算または除算します。要素単位、または行列の乗算を選択し、以下のいずれかを指定してください:
      |  a) 各入力端子に対して * または /。たとえば、**/* は演算 'u1*u2/u3*u4' を実行します。
      |  b) 乗算を行う入力端子の数を指定するスカラー値。たとえば、2 は演算 'u1*u2' を実行します。
      |
      | 1 つの入力端子のみがあり、乗算パラメーターが要素単位 (.*) に設定されている場合、1 つの * または / は、指定した演算を各要素に適用します。しかし、乗算パラメーターが行列 (*) に設定されている場合、1 つの * は行列の乗算を出力し、1 つの / は逆行列を出力します。
      settings: AttributesFormatString=%<Tag>\nOutDataType = %<OutDataTypeStr>
      mask TypeOptions Inputs: Inputs
      mask TypeOptions Multiplication: Multiplication
      mask TypeOptions CollapseMode: CollapseMode
      mask TypeOptions CollapseDim: CollapseDim
      mask TypeOptions SampleTime: SampleTime
      mask TypeOptions InputSameDT: InputSameDT
      mask TypeOptions OutMin: OutMin
      mask TypeOptions OutMax: OutMax
      mask TypeOptions OutDataTypeStr: OutDataTypeStr
      mask TypeOptions LockScale: LockScale
      mask TypeOptions RndMeth: RndMeth
      mask TypeOptions SaturateOnIntegerOverflow: SaturateOnIntegerOverflow
      mask DialogControl Container7 Prompt: メイン
      mask DialogControl Inputs Prompt: 入力数:
      mask DialogControl Multiplication Prompt: 乗算:
      mask DialogControl CollapseMode Prompt: 乗算範囲:
      mask DialogControl CollapseDim Prompt: 次元:
      mask DialogControl SampleTime Prompt: サンプル時間 (継承は -1):
      mask DialogControl Container8 Prompt: 信号属性
      mask DialogControl InputSameDT Prompt: すべての入力が同じデータ型をもつ
      mask DialogControl OutMin Prompt: 出力の最小値:
      mask DialogControl OutMax Prompt: 出力の最大値:
      mask DialogControl OutDataTypeStr Prompt: 出力データ型:
      mask DialogControl LockScale Prompt: 固定小数点ツールによる変更に対して出力データ型の設定をロックする
      mask DialogControl RndMeth Prompt: 整数丸めモード:
      mask DialogControl SaturateOnIntegerOverflow Prompt: 整数オーバーフローで飽和
  Divide3 : Product  Tag=#AMO_Lib  Inputs=*/  CollapseDim=CollapseDim  OutMin=OutMin  OutMax=OutMax  SampleTime=SampleTime  SaturateOnIntegerOverflow=on  RndMeth=Zero  mask{Inputs=*/, Multiplication=Element-wise(.*), CollapseMode=All dimensions, CollapseDim=1, SampleTime=-1, InputSameDT=off, OutMin=[], OutMax=[], OutDataTypeStr=Inherit: Inherit via internal rule, LockScale=off, RndMeth=Zero, SaturateOnIntegerOverflow=on}
      mask prompts: Inputs "Simulink:blkprm_prompts:ProdNumInputs"; Multiplication "Simulink:blkprm_prompts:ProdMultiplication"; CollapseMode "Simulink:blkprm_prompts:ProdOperationType"; CollapseDim "Simulink:blkprm_prompts:ProdOperationDim"; SampleTime "Simulink:blkprm_prompts:AllBlksSampleTime"; InputSameDT "Simulink:blkprm_prompts:InputSameDT"; OutMin "Simulink:blkprm_prompts:OutputDesignMin"; OutMax "Simulink:blkprm_prompts:OutputDesignMax"; OutDataTypeStr "Simulink:blkprm_prompts:OUTPUT_UNIFIEDDATATYPE"; LockScale "Simulink:blkprm_prompts:LockScale"; RndMeth "Simulink:blkprm_prompts:SPP_RndMeth_ID"; SaturateOnIntegerOverflow "Simulink:blkprm_prompts:AllBlksSaturate"
      mask help:
      | 入力を乗算または除算します。要素単位、または行列の乗算を選択し、以下のいずれかを指定してください:
      |  a) 各入力端子に対して * または /。たとえば、**/* は演算 'u1*u2/u3*u4' を実行します。
      |  b) 乗算を行う入力端子の数を指定するスカラー値。たとえば、2 は演算 'u1*u2' を実行します。
      |
      | 1 つの入力端子のみがあり、乗算パラメーターが要素単位 (.*) に設定されている場合、1 つの * または / は、指定した演算を各要素に適用します。しかし、乗算パラメーターが行列 (*) に設定されている場合、1 つの * は行列の乗算を出力し、1 つの / は逆行列を出力します。
      settings: AttributesFormatString=%<Tag>\nOutDataType = %<OutDataTypeStr>
      mask TypeOptions Inputs: Inputs
      mask TypeOptions Multiplication: Multiplication
      mask TypeOptions CollapseMode: CollapseMode
      mask TypeOptions CollapseDim: CollapseDim
      mask TypeOptions SampleTime: SampleTime
      mask TypeOptions InputSameDT: InputSameDT
      mask TypeOptions OutMin: OutMin
      mask TypeOptions OutMax: OutMax
      mask TypeOptions OutDataTypeStr: OutDataTypeStr
      mask TypeOptions LockScale: LockScale
      mask TypeOptions RndMeth: RndMeth
      mask TypeOptions SaturateOnIntegerOverflow: SaturateOnIntegerOverflow
      mask DialogControl Container7 Prompt: メイン
      mask DialogControl Inputs Prompt: 入力数:
      mask DialogControl Multiplication Prompt: 乗算:
      mask DialogControl CollapseMode Prompt: 乗算範囲:
      mask DialogControl CollapseDim Prompt: 次元:
      mask DialogControl SampleTime Prompt: サンプル時間 (継承は -1):
      mask DialogControl Container8 Prompt: 信号属性
      mask DialogControl InputSameDT Prompt: すべての入力が同じデータ型をもつ
      mask DialogControl OutMin Prompt: 出力の最小値:
      mask DialogControl OutMax Prompt: 出力の最大値:
      mask DialogControl OutDataTypeStr Prompt: 出力データ型:
      mask DialogControl LockScale Prompt: 固定小数点ツールによる変更に対して出力データ型の設定をロックする
      mask DialogControl RndMeth Prompt: 整数丸めモード:
      mask DialogControl SaturateOnIntegerOverflow Prompt: 整数オーバーフローで飽和
  Divide4 : Product  Tag=#AMO_Lib  Inputs=*/  CollapseDim=CollapseDim  OutMin=OutMin  OutMax=OutMax  SampleTime=SampleTime  SaturateOnIntegerOverflow=on  RndMeth=Zero  mask{Inputs=*/, Multiplication=Element-wise(.*), CollapseMode=All dimensions, CollapseDim=1, SampleTime=-1, InputSameDT=off, OutMin=[], OutMax=[], OutDataTypeStr=Inherit: Inherit via internal rule, LockScale=off, RndMeth=Zero, SaturateOnIntegerOverflow=on}
      mask prompts: Inputs "Simulink:blkprm_prompts:ProdNumInputs"; Multiplication "Simulink:blkprm_prompts:ProdMultiplication"; CollapseMode "Simulink:blkprm_prompts:ProdOperationType"; CollapseDim "Simulink:blkprm_prompts:ProdOperationDim"; SampleTime "Simulink:blkprm_prompts:AllBlksSampleTime"; InputSameDT "Simulink:blkprm_prompts:InputSameDT"; OutMin "Simulink:blkprm_prompts:OutputDesignMin"; OutMax "Simulink:blkprm_prompts:OutputDesignMax"; OutDataTypeStr "Simulink:blkprm_prompts:OUTPUT_UNIFIEDDATATYPE"; LockScale "Simulink:blkprm_prompts:LockScale"; RndMeth "Simulink:blkprm_prompts:SPP_RndMeth_ID"; SaturateOnIntegerOverflow "Simulink:blkprm_prompts:AllBlksSaturate"
      mask help:
      | 入力を乗算または除算します。要素単位、または行列の乗算を選択し、以下のいずれかを指定してください:
      |  a) 各入力端子に対して * または /。たとえば、**/* は演算 'u1*u2/u3*u4' を実行します。
      |  b) 乗算を行う入力端子の数を指定するスカラー値。たとえば、2 は演算 'u1*u2' を実行します。
      |
      | 1 つの入力端子のみがあり、乗算パラメーターが要素単位 (.*) に設定されている場合、1 つの * または / は、指定した演算を各要素に適用します。しかし、乗算パラメーターが行列 (*) に設定されている場合、1 つの * は行列の乗算を出力し、1 つの / は逆行列を出力します。
      settings: AttributesFormatString=%<Tag>\nOutDataType = %<OutDataTypeStr>
      mask TypeOptions Inputs: Inputs
      mask TypeOptions Multiplication: Multiplication
      mask TypeOptions CollapseMode: CollapseMode
      mask TypeOptions CollapseDim: CollapseDim
      mask TypeOptions SampleTime: SampleTime
      mask TypeOptions InputSameDT: InputSameDT
      mask TypeOptions OutMin: OutMin
      mask TypeOptions OutMax: OutMax
      mask TypeOptions OutDataTypeStr: OutDataTypeStr
      mask TypeOptions LockScale: LockScale
      mask TypeOptions RndMeth: RndMeth
      mask TypeOptions SaturateOnIntegerOverflow: SaturateOnIntegerOverflow
      mask DialogControl Container7 Prompt: メイン
      mask DialogControl Inputs Prompt: 入力数:
      mask DialogControl Multiplication Prompt: 乗算:
      mask DialogControl CollapseMode Prompt: 乗算範囲:
      mask DialogControl CollapseDim Prompt: 次元:
      mask DialogControl SampleTime Prompt: サンプル時間 (継承は -1):
      mask DialogControl Container8 Prompt: 信号属性
      mask DialogControl InputSameDT Prompt: すべての入力が同じデータ型をもつ
      mask DialogControl OutMin Prompt: 出力の最小値:
      mask DialogControl OutMax Prompt: 出力の最大値:
      mask DialogControl OutDataTypeStr Prompt: 出力データ型:
      mask DialogControl LockScale Prompt: 固定小数点ツールによる変更に対して出力データ型の設定をロックする
      mask DialogControl RndMeth Prompt: 整数丸めモード:
      mask DialogControl SaturateOnIntegerOverflow Prompt: 整数オーバーフローで飽和
  Divide5 : Product  Tag=#AMO_Lib  Inputs=*/  CollapseDim=CollapseDim  OutMin=OutMin  OutMax=OutMax  SampleTime=SampleTime  SaturateOnIntegerOverflow=on  RndMeth=Zero  mask{Inputs=*/, Multiplication=Element-wise(.*), CollapseMode=All dimensions, CollapseDim=1, SampleTime=-1, InputSameDT=off, OutMin=[], OutMax=[], OutDataTypeStr=Inherit: Inherit via internal rule, LockScale=off, RndMeth=Zero, SaturateOnIntegerOverflow=on}
      mask prompts: Inputs "Simulink:blkprm_prompts:ProdNumInputs"; Multiplication "Simulink:blkprm_prompts:ProdMultiplication"; CollapseMode "Simulink:blkprm_prompts:ProdOperationType"; CollapseDim "Simulink:blkprm_prompts:ProdOperationDim"; SampleTime "Simulink:blkprm_prompts:AllBlksSampleTime"; InputSameDT "Simulink:blkprm_prompts:InputSameDT"; OutMin "Simulink:blkprm_prompts:OutputDesignMin"; OutMax "Simulink:blkprm_prompts:OutputDesignMax"; OutDataTypeStr "Simulink:blkprm_prompts:OUTPUT_UNIFIEDDATATYPE"; LockScale "Simulink:blkprm_prompts:LockScale"; RndMeth "Simulink:blkprm_prompts:SPP_RndMeth_ID"; SaturateOnIntegerOverflow "Simulink:blkprm_prompts:AllBlksSaturate"
      mask help:
      | 入力を乗算または除算します。要素単位、または行列の乗算を選択し、以下のいずれかを指定してください:
      |  a) 各入力端子に対して * または /。たとえば、**/* は演算 'u1*u2/u3*u4' を実行します。
      |  b) 乗算を行う入力端子の数を指定するスカラー値。たとえば、2 は演算 'u1*u2' を実行します。
      |
      | 1 つの入力端子のみがあり、乗算パラメーターが要素単位 (.*) に設定されている場合、1 つの * または / は、指定した演算を各要素に適用します。しかし、乗算パラメーターが行列 (*) に設定されている場合、1 つの * は行列の乗算を出力し、1 つの / は逆行列を出力します。
      settings: AttributesFormatString=%<Tag>\nOutDataType = %<OutDataTypeStr>
      mask TypeOptions Inputs: Inputs
      mask TypeOptions Multiplication: Multiplication
      mask TypeOptions CollapseMode: CollapseMode
      mask TypeOptions CollapseDim: CollapseDim
      mask TypeOptions SampleTime: SampleTime
      mask TypeOptions InputSameDT: InputSameDT
      mask TypeOptions OutMin: OutMin
      mask TypeOptions OutMax: OutMax
      mask TypeOptions OutDataTypeStr: OutDataTypeStr
      mask TypeOptions LockScale: LockScale
      mask TypeOptions RndMeth: RndMeth
      mask TypeOptions SaturateOnIntegerOverflow: SaturateOnIntegerOverflow
      mask DialogControl Container7 Prompt: メイン
      mask DialogControl Inputs Prompt: 入力数:
      mask DialogControl Multiplication Prompt: 乗算:
      mask DialogControl CollapseMode Prompt: 乗算範囲:
      mask DialogControl CollapseDim Prompt: 次元:
      mask DialogControl SampleTime Prompt: サンプル時間 (継承は -1):
      mask DialogControl Container8 Prompt: 信号属性
      mask DialogControl InputSameDT Prompt: すべての入力が同じデータ型をもつ
      mask DialogControl OutMin Prompt: 出力の最小値:
      mask DialogControl OutMax Prompt: 出力の最大値:
      mask DialogControl OutDataTypeStr Prompt: 出力データ型:
      mask DialogControl LockScale Prompt: 固定小数点ツールによる変更に対して出力データ型の設定をロックする
      mask DialogControl RndMeth Prompt: 整数丸めモード:
      mask DialogControl SaturateOnIntegerOverflow Prompt: 整数オーバーフローで飽和
  Divide6 : Product  Tag=#AMO_Lib  Inputs=*/  CollapseDim=CollapseDim  OutMin=OutMin  OutMax=OutMax  SampleTime=SampleTime  SaturateOnIntegerOverflow=on  RndMeth=Zero  mask{Inputs=*/, Multiplication=Element-wise(.*), CollapseMode=All dimensions, CollapseDim=1, SampleTime=-1, InputSameDT=off, OutMin=[], OutMax=[], OutDataTypeStr=Inherit: Inherit via internal rule, LockScale=off, RndMeth=Zero, SaturateOnIntegerOverflow=on}
      mask prompts: Inputs "Simulink:blkprm_prompts:ProdNumInputs"; Multiplication "Simulink:blkprm_prompts:ProdMultiplication"; CollapseMode "Simulink:blkprm_prompts:ProdOperationType"; CollapseDim "Simulink:blkprm_prompts:ProdOperationDim"; SampleTime "Simulink:blkprm_prompts:AllBlksSampleTime"; InputSameDT "Simulink:blkprm_prompts:InputSameDT"; OutMin "Simulink:blkprm_prompts:OutputDesignMin"; OutMax "Simulink:blkprm_prompts:OutputDesignMax"; OutDataTypeStr "Simulink:blkprm_prompts:OUTPUT_UNIFIEDDATATYPE"; LockScale "Simulink:blkprm_prompts:LockScale"; RndMeth "Simulink:blkprm_prompts:SPP_RndMeth_ID"; SaturateOnIntegerOverflow "Simulink:blkprm_prompts:AllBlksSaturate"
      mask help:
      | 入力を乗算または除算します。要素単位、または行列の乗算を選択し、以下のいずれかを指定してください:
      |  a) 各入力端子に対して * または /。たとえば、**/* は演算 'u1*u2/u3*u4' を実行します。
      |  b) 乗算を行う入力端子の数を指定するスカラー値。たとえば、2 は演算 'u1*u2' を実行します。
      |
      | 1 つの入力端子のみがあり、乗算パラメーターが要素単位 (.*) に設定されている場合、1 つの * または / は、指定した演算を各要素に適用します。しかし、乗算パラメーターが行列 (*) に設定されている場合、1 つの * は行列の乗算を出力し、1 つの / は逆行列を出力します。
      settings: AttributesFormatString=%<Tag>\nOutDataType = %<OutDataTypeStr>
      mask TypeOptions Inputs: Inputs
      mask TypeOptions Multiplication: Multiplication
      mask TypeOptions CollapseMode: CollapseMode
      mask TypeOptions CollapseDim: CollapseDim
      mask TypeOptions SampleTime: SampleTime
      mask TypeOptions InputSameDT: InputSameDT
      mask TypeOptions OutMin: OutMin
      mask TypeOptions OutMax: OutMax
      mask TypeOptions OutDataTypeStr: OutDataTypeStr
      mask TypeOptions LockScale: LockScale
      mask TypeOptions RndMeth: RndMeth
      mask TypeOptions SaturateOnIntegerOverflow: SaturateOnIntegerOverflow
      mask DialogControl Container7 Prompt: メイン
      mask DialogControl Inputs Prompt: 入力数:
      mask DialogControl Multiplication Prompt: 乗算:
      mask DialogControl CollapseMode Prompt: 乗算範囲:
      mask DialogControl CollapseDim Prompt: 次元:
      mask DialogControl SampleTime Prompt: サンプル時間 (継承は -1):
      mask DialogControl Container8 Prompt: 信号属性
      mask DialogControl InputSameDT Prompt: すべての入力が同じデータ型をもつ
      mask DialogControl OutMin Prompt: 出力の最小値:
      mask DialogControl OutMax Prompt: 出力の最大値:
      mask DialogControl OutDataTypeStr Prompt: 出力データ型:
      mask DialogControl LockScale Prompt: 固定小数点ツールによる変更に対して出力データ型の設定をロックする
      mask DialogControl RndMeth Prompt: 整数丸めモード:
      mask DialogControl SaturateOnIntegerOverflow Prompt: 整数オーバーフローで飽和
  Event Listener : EventListener  DisableCoverage=on  EventType=Reset  EventName=JINIT_rcv_info10m
  Saturation : Saturate  Tag=#AMO_Lib  UpperLimit=UpperLimit  LowerLimit=LowerLimit  SampleTime=SampleTime  OutMin=OutMin  OutMax=OutMax  RndMeth=Zero  mask{UpperLimit=360000, LowerLimit=0, LinearizeAsGain=on, ZeroCross=on, SampleTime=-1, OutMin=[], OutMax=[], OutDataTypeStr=Inherit: Same as input, LockScale=off, RndMeth=Zero}
      mask prompts: UpperLimit "Simulink:blkprm_prompts:SaturateUpLim"; LowerLimit "Simulink:blkprm_prompts:SaturateLowLim"; LinearizeAsGain "Simulink:blkprm_prompts:LinearizeAsGain"; ZeroCross "Simulink:blkprm_prompts:AllBlksEnableZC"; SampleTime "Simulink:blkprm_prompts:AllBlksSampleTime"; OutMin "Simulink:blkprm_prompts:OutputDesignMin"; OutMax "Simulink:blkprm_prompts:OutputDesignMax"; OutDataTypeStr "Simulink:blkprm_prompts:OUTPUT_UNIFIEDDATATYPE"; LockScale "Simulink:blkprm_prompts:LockScale"; RndMeth "Simulink:blkprm_prompts:SPP_RndMeth_ID"
      mask help: 入力信号を上限と下限の飽和値に制約します。
      settings: AttributesFormatString=%<Tag>\n%<LowerLimit> - %<UpperLimit>\nOutDataType = %<OutDataTypeStr>
      mask TypeOptions UpperLimit: UpperLimit
      mask TypeOptions LowerLimit: LowerLimit
      mask TypeOptions LinearizeAsGain: LinearizeAsGain
      mask TypeOptions ZeroCross: ZeroCross
      mask TypeOptions SampleTime: SampleTime
      mask TypeOptions OutMin: OutMin
      mask TypeOptions OutMax: OutMax
      mask TypeOptions OutDataTypeStr: OutDataTypeStr
      mask TypeOptions LockScale: LockScale
      mask TypeOptions RndMeth: RndMeth
      mask DialogControl Container4 Prompt: メイン
      mask DialogControl UpperLimit Prompt: 上限:
      mask DialogControl LowerLimit Prompt: 下限:
      mask DialogControl LinearizeAsGain Prompt: 線形化時にゲインとして扱う
      mask DialogControl ZeroCross Prompt: ゼロクロッシング検出を有効にする
      mask DialogControl SampleTime Prompt: サンプル時間 (継承は -1):
      mask DialogControl Container5 Prompt: 信号属性
      mask DialogControl OutMin Prompt: 出力の最小値:
      mask DialogControl OutMax Prompt: 出力の最大値:
      mask DialogControl OutDataTypeStr Prompt: 出力データ型:
      mask DialogControl LockScale Prompt: 固定小数点ツールによる変更に対して出力データ型の設定をロックする
      mask DialogControl RndMeth Prompt: 整数丸めモード:
  Saturation1 : Saturate  Tag=#AMO_Lib  UpperLimit=UpperLimit  LowerLimit=LowerLimit  SampleTime=SampleTime  OutMin=OutMin  OutMax=OutMax  RndMeth=Zero  mask{UpperLimit=100, LowerLimit=-100, LinearizeAsGain=on, ZeroCross=on, SampleTime=-1, OutMin=[], OutMax=[], OutDataTypeStr=Inherit: Same as input, LockScale=off, RndMeth=Zero}
      mask prompts: UpperLimit "Simulink:blkprm_prompts:SaturateUpLim"; LowerLimit "Simulink:blkprm_prompts:SaturateLowLim"; LinearizeAsGain "Simulink:blkprm_prompts:LinearizeAsGain"; ZeroCross "Simulink:blkprm_prompts:AllBlksEnableZC"; SampleTime "Simulink:blkprm_prompts:AllBlksSampleTime"; OutMin "Simulink:blkprm_prompts:OutputDesignMin"; OutMax "Simulink:blkprm_prompts:OutputDesignMax"; OutDataTypeStr "Simulink:blkprm_prompts:OUTPUT_UNIFIEDDATATYPE"; LockScale "Simulink:blkprm_prompts:LockScale"; RndMeth "Simulink:blkprm_prompts:SPP_RndMeth_ID"
      mask help: 入力信号を上限と下限の飽和値に制約します。
      settings: AttributesFormatString=%<Tag>\n%<LowerLimit> - %<UpperLimit>\nOutDataType = %<OutDataTypeStr>
      mask TypeOptions UpperLimit: UpperLimit
      mask TypeOptions LowerLimit: LowerLimit
      mask TypeOptions LinearizeAsGain: LinearizeAsGain
      mask TypeOptions ZeroCross: ZeroCross
      mask TypeOptions SampleTime: SampleTime
      mask TypeOptions OutMin: OutMin
      mask TypeOptions OutMax: OutMax
      mask TypeOptions OutDataTypeStr: OutDataTypeStr
      mask TypeOptions LockScale: LockScale
      mask TypeOptions RndMeth: RndMeth
      mask DialogControl Container4 Prompt: メイン
      mask DialogControl UpperLimit Prompt: 上限:
      mask DialogControl LowerLimit Prompt: 下限:
      mask DialogControl LinearizeAsGain Prompt: 線形化時にゲインとして扱う
      mask DialogControl ZeroCross Prompt: ゼロクロッシング検出を有効にする
      mask DialogControl SampleTime Prompt: サンプル時間 (継承は -1):
      mask DialogControl Container5 Prompt: 信号属性
      mask DialogControl OutMin Prompt: 出力の最小値:
      mask DialogControl OutMax Prompt: 出力の最大値:
      mask DialogControl OutDataTypeStr Prompt: 出力データ型:
      mask DialogControl LockScale Prompt: 固定小数点ツールによる変更に対して出力データ型の設定をロックする
      mask DialogControl RndMeth Prompt: 整数丸めモード:
  Saturation2 : Saturate  Tag=#AMO_Lib  UpperLimit=UpperLimit  LowerLimit=LowerLimit  SampleTime=SampleTime  OutMin=OutMin  OutMax=OutMax  RndMeth=Zero  mask{UpperLimit=100, LowerLimit=-100, LinearizeAsGain=on, ZeroCross=on, SampleTime=-1, OutMin=[], OutMax=[], OutDataTypeStr=Inherit: Same as input, LockScale=off, RndMeth=Zero}
      mask prompts: UpperLimit "Simulink:blkprm_prompts:SaturateUpLim"; LowerLimit "Simulink:blkprm_prompts:SaturateLowLim"; LinearizeAsGain "Simulink:blkprm_prompts:LinearizeAsGain"; ZeroCross "Simulink:blkprm_prompts:AllBlksEnableZC"; SampleTime "Simulink:blkprm_prompts:AllBlksSampleTime"; OutMin "Simulink:blkprm_prompts:OutputDesignMin"; OutMax "Simulink:blkprm_prompts:OutputDesignMax"; OutDataTypeStr "Simulink:blkprm_prompts:OUTPUT_UNIFIEDDATATYPE"; LockScale "Simulink:blkprm_prompts:LockScale"; RndMeth "Simulink:blkprm_prompts:SPP_RndMeth_ID"
      mask help: 入力信号を上限と下限の飽和値に制約します。
      settings: AttributesFormatString=%<Tag>\n%<LowerLimit> - %<UpperLimit>\nOutDataType = %<OutDataTypeStr>
      mask TypeOptions UpperLimit: UpperLimit
      mask TypeOptions LowerLimit: LowerLimit
      mask TypeOptions LinearizeAsGain: LinearizeAsGain
      mask TypeOptions ZeroCross: ZeroCross
      mask TypeOptions SampleTime: SampleTime
      mask TypeOptions OutMin: OutMin
      mask TypeOptions OutMax: OutMax
      mask TypeOptions OutDataTypeStr: OutDataTypeStr
      mask TypeOptions LockScale: LockScale
      mask TypeOptions RndMeth: RndMeth
      mask DialogControl Container4 Prompt: メイン
      mask DialogControl UpperLimit Prompt: 上限:
      mask DialogControl LowerLimit Prompt: 下限:
      mask DialogControl LinearizeAsGain Prompt: 線形化時にゲインとして扱う
      mask DialogControl ZeroCross Prompt: ゼロクロッシング検出を有効にする
      mask DialogControl SampleTime Prompt: サンプル時間 (継承は -1):
      mask DialogControl Container5 Prompt: 信号属性
      mask DialogControl OutMin Prompt: 出力の最小値:
      mask DialogControl OutMax Prompt: 出力の最大値:
      mask DialogControl OutDataTypeStr Prompt: 出力データ型:
      mask DialogControl LockScale Prompt: 固定小数点ツールによる変更に対して出力データ型の設定をロックする
      mask DialogControl RndMeth Prompt: 整数丸めモード:
  State Writer : StateWriter  StateOwnerBlock=../../Simulink Function/v_bc_pl_s
  State Writer1 : StateWriter  StateOwnerBlock=../../Simulink Function/as_bcbsmin_pl_s
  State Writer2 : StateWriter  StateOwnerBlock=../../Simulink Function/i_bat_10m_pl_s
  State Writer3 : StateWriter  StateOwnerBlock=../../Simulink Function/t_bmax_pl_s
  State Writer4 : StateWriter  StateOwnerBlock=../../Simulink Function/t_bmin_pl_s
  State Writer5 : StateWriter  StateOwnerBlock=../../Simulink Function/v_bcocvmax_pl_s
  State Writer6 : StateWriter  StateOwnerBlock=../../Simulink Function/v_bcocvmin_pl_s
  State Writer7 : StateWriter  StateOwnerBlock=../../Simulink Function/sc_bcmax_pl
  State Writer8 : StateWriter  StateOwnerBlock=../../Simulink Function/sc_bcmin_pl
  State Writer9 : StateWriter  StateOwnerBlock=../../Simulink Function/v_bcmax_pl
  asbcbaseini_C : Constant  Tag=#AMO_Lib  Value=asbcbaseini_C
      settings: AttributesFormatString=%<Tag>\nOutDataType = %<OutDataTypeStr>
  ibatini_C : Constant  Tag=#AMO_Lib  Value=ibatini_C
      settings: AttributesFormatString=%<Tag>\nOutDataType = %<OutDataTypeStr>
  scsocini_C : Constant  Tag=#AMO_Lib  Value=scsocini_C
      settings: AttributesFormatString=%<Tag>\nOutDataType = %<OutDataTypeStr>
  t_bmaxini_C : Constant  Tag=#AMO_Lib  Value=t_bmaxini_C
      settings: AttributesFormatString=%<Tag>\nOutDataType = %<OutDataTypeStr>
  t_bminini_C : Constant  Tag=#AMO_Lib  Value=t_bminini_C
      settings: AttributesFormatString=%<Tag>\nOutDataType = %<OutDataTypeStr>
  v_bcini_C : Constant  Tag=#AMO_Lib  Value=v_bcini_C
      settings: AttributesFormatString=%<Tag>\nOutDataType = %<OutDataTypeStr>
  v_bcmaxini_C : Constant  Tag=#AMO_Lib  Value=v_bcmaxini_C
      settings: AttributesFormatString=%<Tag>\nOutDataType = %<OutDataTypeStr>
  wires:
  Data Type Conversion/1 -> Divide/1
  Constant/1 -> Divide/2
  Divide/1 -> Data Type Conversion1/1
  Data Type Conversion1/1 -> State Writer/1
  asbcbaseini_C/1 -> Data Type Conversion2/1
  Data Type Conversion2/1 -> Divide1/1
  Constant1/1 -> Divide1/2
  Divide1/1 -> Data Type Conversion3/1
  Data Type Conversion3/1 -> Saturation/1
  Saturation/1 -> State Writer1/1
  Divide2/1 -> Data Type Conversion5/1
  Data Type Conversion5/1 -> State Writer2/1
  Constant2/1 -> Divide2/2
  Data Type Conversion4/1 -> Divide2/1
  ibatini_C/1 -> Data Type Conversion4/1
  Data Type Conversion7/1 -> Saturation1/1
  Divide3/1 -> Data Type Conversion7/1
  Saturation1/1 -> State Writer3/1
  Constant3/1 -> Divide3/2
  Data Type Conversion6/1 -> Divide3/1
  t_bmaxini_C/1 -> Data Type Conversion6/1
  t_bminini_C/1 -> Data Type Conversion8/1
  Data Type Conversion9/1 -> Saturation2/1
  Data Type Conversion8/1 -> Divide4/1
  Constant4/1 -> Divide4/2
  Divide4/1 -> Data Type Conversion9/1
  Saturation2/1 -> State Writer4/1
  Data Type Conversion11/1 -> State Writer5/1
  Data Type Conversion10/1 -> Divide5/1
  Constant5/1 -> Divide5/2
  Divide5/1 -> Data Type Conversion11/1
  Data Type Conversion13/1 -> State Writer6/1
  Data Type Conversion12/1 -> Divide6/1
  v_bcini_C/1 -> Data Type Conversion/1, Data Type Conversion12/1, Data Type Conversion10/1
  Constant6/1 -> Divide6/2
  Divide6/1 -> Data Type Conversion13/1
  v_bcmaxini_C/1 -> State Writer9/1
  scsocini_C/1 -> State Writer8/1, State Writer7/1
